simulink model "rev3_PEM"  (R2024a)
settings: Solver=VariableStepAuto  StartTime=0.0  StopTime=10.0  RelTol=1e-3
libraries: spsParallelRLCBranchLib x5
settings Model: Creator=ADMIN  LastModifiedBy=ADMIN

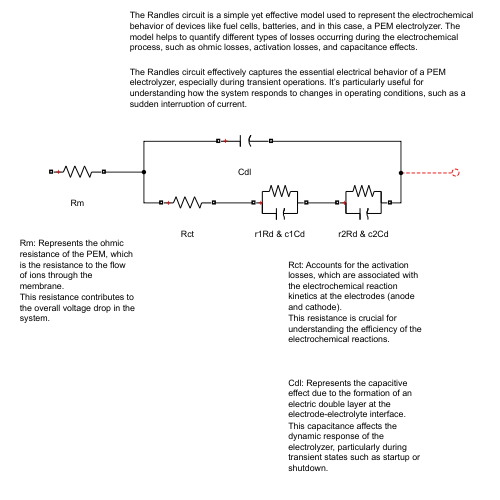
[thumbnail: Simulink's stored preview of the top-level diagram]
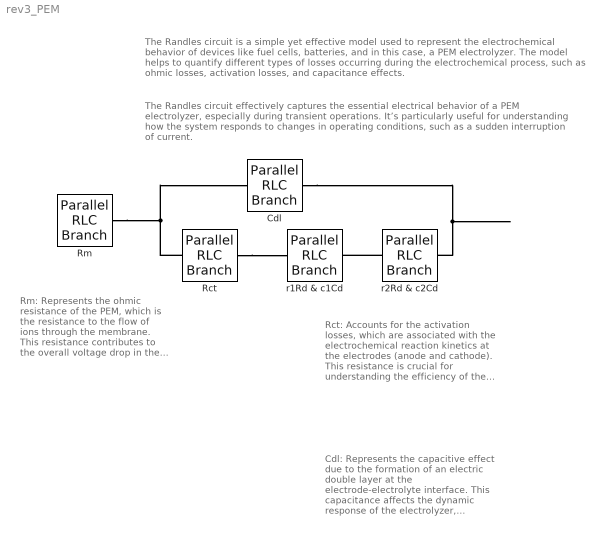
== system rev3_PEM ==
  note: The Randles circuit effectively captures the essential electrical behavior of a PEM electrolyzer, especially during transient operations. It’s particularly useful for understanding how the system responds to changes in operating conditions, such as a sudden interruption of current.
  note: Cdl: Represents the capacitive effect due to the formation of an electric double layer at the electrode-electrolyte interface.
      | This capacitance affects the dynamic response of the electrolyzer, particularly during transient states such as startup or shutdown.
  note: Rct: Accounts for the activation losses, which are associated with the electrochemical reaction kinetics at the electrodes (anode and cathode).
      | This resistance is crucial for understanding the efficiency of the electrochemical reactions.
  note: Rm: Represents the ohmic resistance of the PEM, which is the resistance to the flow of ions through the membrane.
      | This resistance contributes to the overall voltage drop in the system.
  note: The Randles circuit is a simple yet effective model used to represent the electrochemical behavior of devices like fuel cells, batteries, and in this case, a PEM electrolyzer. The model helps to quantify different types of losses occurring during the electrochemical process, such as ohmic losses, activation losses, and capacitance effects.
  Cdl : spsParallelRLCBranchLib/Parallel RLC Branch  LConnTagsString=a  RConnTagsString=__new0  BranchType=C  Resistance=1  Inductance=1e-3  SetiL0=off  InitialCurrent=0  Capacitance=1e-6  Setx0=off  InitialVoltage=0  Measurements=None
  Rct : spsParallelRLCBranchLib/Parallel RLC Branch  LConnTagsString=a  RConnTagsString=__new0  BranchType=R  Resistance=1  Inductance=1e-3  SetiL0=off  InitialCurrent=0  Capacitance=1e-6  Setx0=off  InitialVoltage=0  Measurements=None
  Rm : spsParallelRLCBranchLib/Parallel RLC Branch  LConnTagsString=a  RConnTagsString=__new0  BranchType=R  Resistance=1  Inductance=1e-3  SetiL0=off  InitialCurrent=0  Capacitance=1e-6  Setx0=off  InitialVoltage=0  Measurements=None
  r1Rd & c1Cd : spsParallelRLCBranchLib/Parallel RLC Branch  LConnTagsString=a  RConnTagsString=__new0  BranchType=RC  Resistance=1  Inductance=1e-3  SetiL0=off  InitialCurrent=0  Capacitance=1e-6  Setx0=off  InitialVoltage=0  Measurements=None
  r2Rd & c2Cd : spsParallelRLCBranchLib/Parallel RLC Branch  LConnTagsString=a  RConnTagsString=__new0  BranchType=RC  Resistance=1  Inductance=1e-3  SetiL0=off  InitialCurrent=0  Capacitance=1e-6  Setx0=off  InitialVoltage=0  Measurements=None
  connections:
  Rct/RConn1 -- r1Rd & c1Cd/LConn1
  r2Rd & c2Cd/LConn1 -- r1Rd & c1Cd/RConn1
  Rm/RConn1 -- Cdl/LConn1 -- Rct/LConn1
  Cdl/RConn1 -- r2Rd & c2Cd/RConn1
